simulink model "AeroDynamicForce"  (R2021a)
settings: Solver=VariableStepAuto  StartTime=0.0  StopTime=10.0  RelTol=1e-3
settings Model: Creator=gopin  LastModifiedBy=gopin

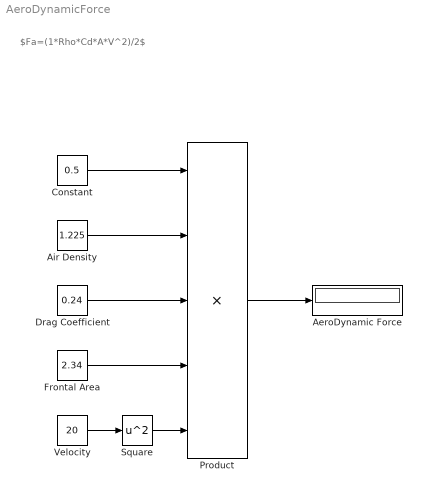
== system AeroDynamicForce ==
  note: $Fa=(1*Rho*Cd*A*V^2)/2$
  AeroDynamic Force : Display
  Air Density : Constant  Value=1.225
  Constant : Constant  Value=0.5
  Drag Coefficient : Constant  Value=0.24
  Frontal Area : Constant  Value=2.34
  Product : Product  Inputs=5
  Square : Math  Operator=square  SaturateOnIntegerOverflow=on
  Velocity : Constant  Value=20
  wires:
  Constant/1 -> Product/1
  Air Density/1 -> Product/2
  Drag Coefficient/1 -> Product/3
  Frontal Area/1 -> Product/4
  Product/1 -> AeroDynamic Force/1
  Velocity/1 -> Square/1
  Square/1 -> Product/5
